simulink model "ball_beam_sim"  (R2021a)
settings: Solver=ode4  StartTime=0.0  StopTime=30  FixedStep=1e-3  RelTol=1e-3
values from neighbouring files (symbols this model uses):
  g = 9.81    [parameters_definition.m]
  J = 9.99e-6    (= 9.99e-06)    [parameters_definition.m]
  m = 0.11    [parameters_definition.m]
  R = 0.015    [parameters_definition.m]
settings Model: Creator=Luis Costa  LastModifiedBy=Luis

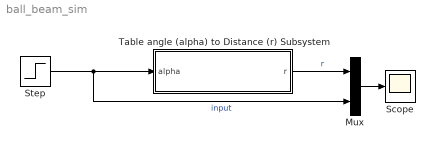
== system ball_beam_sim ==
  Mux : Mux  Inputs=2
  Scope : Scope
  Step : Step  After=0.001  SampleTime=0
  Table angle (alpha) to Distance (r) Subsystem : Subsystem
  wires:
  Table angle (alpha) to Distance (r) Subsystem/1(r) -> Mux/1  "r"
  Mux/1 -> Scope/1
  Step/1 -> Mux/2, Table angle (alpha) to Distance (r) Subsystem/1(alpha)  "input"

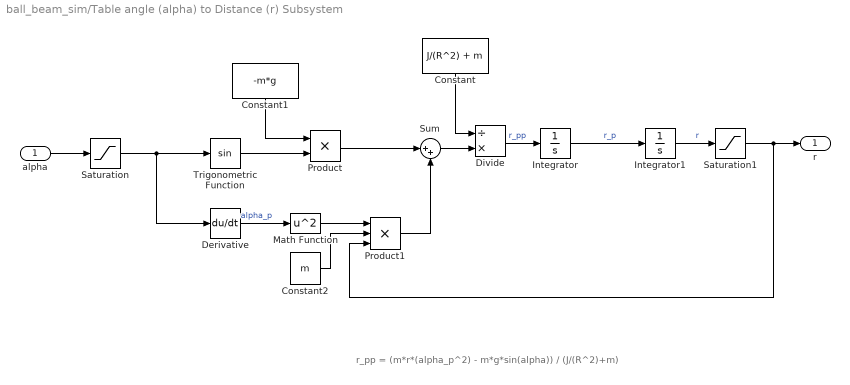
== system ball_beam_sim/Table angle (alpha) to Distance (r) Subsystem ==
  note: r_pp = (m*r*(alpha_p^2) - m*g*sin(alpha)) / (J/(R^2)+m)
  alpha : Inport
  Constant : Constant  Value=J/(R^2) + m
  Constant1 : Constant  Value=-m*g
  Constant2 : Constant  Value=m
  Derivative : Derivative
  Divide : Product  Inputs=/*
  Integrator : Integrator
  Integrator1 : Integrator  InitialCondition=0.08
  Math Function : Math  Operator=square  SaturateOnIntegerOverflow=on
  Product : Product
  Product1 : Product  Inputs=3
  Saturation : Saturate  UpperLimit=0.263  LowerLimit=-0.2
  Saturation1 : Saturate  UpperLimit=0.3  LowerLimit=0.04
  Sum : Sum  Inputs=|++
  Trigonometric Function : Trigonometry
  r : Outport
  wires:
  Constant1/1 -> Product/1
  Constant/1 -> Divide/1
  alpha/1 -> Saturation/1
  Integrator/1 -> Integrator1/1  "r_p"
  Math Function/1 -> Product1/1
  Sum/1 -> Divide/2
  Trigonometric Function/1 -> Product/2
  Constant2/1 -> Product1/2
  Derivative/1 -> Math Function/1  "alpha_p"
  Product/1 -> Sum/1
  Product1/1 -> Sum/2
  Divide/1 -> Integrator/1  "r_pp"
  Saturation/1 -> Derivative/1, Trigonometric Function/1
  Integrator1/1 -> Saturation1/1  "r"
  Saturation1/1 -> Product1/3, r/1
